simulink model "SMPI"  (R2020a)
settings: Solver=VariableStepAuto  StartTime=0.0  StopTime=15  RelTol=1e-3
settings Model: Creator=alfan  LastModifiedBy=alfan

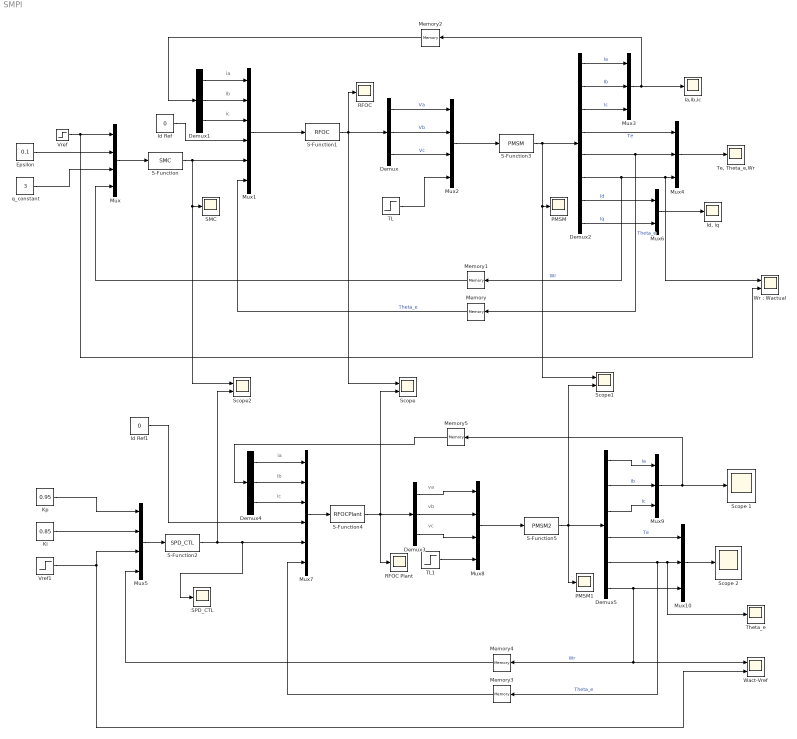
== system SMPI ==
  note: ia
  note: ib
  note: ic
  note: ia
  note: vc
  note: ib
  note: vb
  note: ic
  note: va
  Demux{,1,3..4} (4 alike) : Demux  Outputs=3
  Demux2 : Demux  Outputs=8
  Demux5 : Demux  Outputs=6
  Epsilon : Constant  Value=0.1
  Ia,ib,ic : Scope
  Id Ref : Constant  Value=0
  Id Ref1 : Constant  Value=0
  "Id, iq" : Scope
  Ki : Constant  Value=0.85
  Kp : Constant  Value=0.95
  Memory : Memory  InheritSampleTime=on
  Memory{1..2,4..5} (4 alike) : Memory
  Memory3 : Memory  InheritSampleTime=on
  Mux{,2,5,8} (4 alike) : Mux
  Mux1 : Mux  Inputs=6
  Mux{3..4,9..10} (4 alike) : Mux  Inputs=3
  Mux6 : Mux  Inputs=2
  Mux7 : Mux  Inputs=6
  PMSM : Scope
  PMSM1 : Scope
  RFOC : Scope
  RFOC Plant : Scope
  S-Function : S-Function  FunctionName=SMC  SFunctionDeploymentMode=off  EnableBusSupport=off
  S-Function1 : S-Function  FunctionName=RFOC  SFunctionDeploymentMode=off  EnableBusSupport=off
  S-Function2 : S-Function  FunctionName=SPD_CTL  SFunctionDeploymentMode=off  EnableBusSupport=off
  S-Function3 : S-Function  FunctionName=PMSM  SFunctionDeploymentMode=off  EnableBusSupport=off
  S-Function4 : S-Function  FunctionName=RFOCPlant  SFunctionDeploymentMode=off  EnableBusSupport=off
  S-Function5 : S-Function  FunctionName=PMSM2  SFunctionDeploymentMode=off  EnableBusSupport=off
  SMC : Scope
  SPD_CTL : Scope
  Scope : Scope  NumInputPorts=2
  Scope 1 : Scope
  Scope 2 : Scope
  Scope1 : Scope  NumInputPorts=2
  Scope2 : Scope  NumInputPorts=2
  TL : Step  SampleTime=0
  TL1 : Step  After=3  SampleTime=0
  "Te, Theta_e,Wr" : Scope
  Theta_e : Scope
  Vref : Step  After=20  SampleTime=0
  Vref1 : Step  Time=3  After=10  SampleTime=0
  Wact-Vref : Scope  NumInputPorts=2
  "Wr : Wactual" : Scope  NumInputPorts=2
  q_constant : Constant  Value=3
  wires:
  Mux/1 -> S-Function/1
  S-Function/1 -> Scope2/1, SMC/1, Mux1/5
  Mux1/1 -> S-Function1/1
  S-Function1/1 -> Scope/1, RFOC/1, Demux/1
  TL/1 -> Mux2/4
  Demux/3 -> Mux2/3  "Vc"
  Demux/2 -> Mux2/2  "Vb"
  Demux/1 -> Mux2/1  "Va"
  Demux1/1 -> Mux1/1
  Demux1/2 -> Mux1/2
  Demux1/3 -> Mux1/3
  Mux2/1 -> S-Function3/1
  S-Function3/1 -> Scope1/1, PMSM/1, Demux2/1
  Demux2/5 -> Memory/1, Mux4/2  "Theta_e"
  Demux2/1 -> Mux3/1  "Ia"
  Demux2/2 -> Mux3/2  "Ib"
  Demux2/3 -> Mux3/3  "Ic"
  Mux3/1 -> Ia,ib,ic/1, Memory2/1
  Memory2/1 -> Demux1/1
  Demux2/4 -> Mux4/1  "Te"
  Demux2/6 -> Memory1/1, "Wr : Wactual"/1, Mux4/3  "Wr"
  Memory/1 -> Mux1/6  "Theta_e"
  Id Ref/1 -> Mux1/4
  Demux2/7 -> Mux6/1  "Id"
  Demux2/8 -> Mux6/2  "Iq"
  Memory1/1 -> Mux/4
  Epsilon/1 -> Mux/2
  q_constant/1 -> Mux/3
  Mux4/1 -> "Te, Theta_e,Wr"/1
  Mux6/1 -> "Id, iq"/1
  Vref/1 -> Mux/1, "Wr : Wactual"/2
  Memory4/1 -> Mux5/4
  Demux5/5 -> Memory3/1, Theta_e/1, Mux10/2  "Theta_e"
  Mux8/1 -> S-Function5/1
  Memory5/1 -> Demux4/1
  Demux3/3 -> Mux8/3
  Demux5/3 -> Mux9/3  "Ic"
  Demux5/1 -> Mux9/1  "Ia"
  Mux9/1 -> Memory5/1, Scope 1/1
  Memory3/1 -> Mux7/6
  Id Ref1/1 -> Mux7/4
  Ki/1 -> Mux5/2
  Demux5/6 -> Wact-Vref/1, Memory4/1, Mux10/3  "Wr"
  Vref1/1 -> Wact-Vref/2, Mux5/3
  Demux3/1 -> Mux8/1
  Demux5/2 -> Mux9/2  "Ib"
  Demux4/3 -> Mux7/3
  S-Function5/1 -> Scope1/2, PMSM1/1, Demux5/1
  Demux5/4 -> Mux10/1  "Te"
  S-Function4/1 -> Scope/2, RFOC Plant/1, Demux3/1
  S-Function2/1 -> Scope2/2, SPD_CTL/1, Mux7/5
  Mux5/1 -> S-Function2/1
  Mux10/1 -> Scope 2/1
  Demux4/2 -> Mux7/2
  Mux7/1 -> S-Function4/1
  TL1/1 -> Mux8/4
  Demux4/1 -> Mux7/1
  Kp/1 -> Mux5/1
  Demux3/2 -> Mux8/2
